simulink model "TermProject_Rectifier"  (R2019a)
settings: Solver=FixedStepDiscrete  StartTime=0.0  StopTime=1  RelTol=1e-3
libraries: powerlib x22, eeGeneralControl x4
settings Model: Creator=ryusl  LastModifiedBy=ryusl

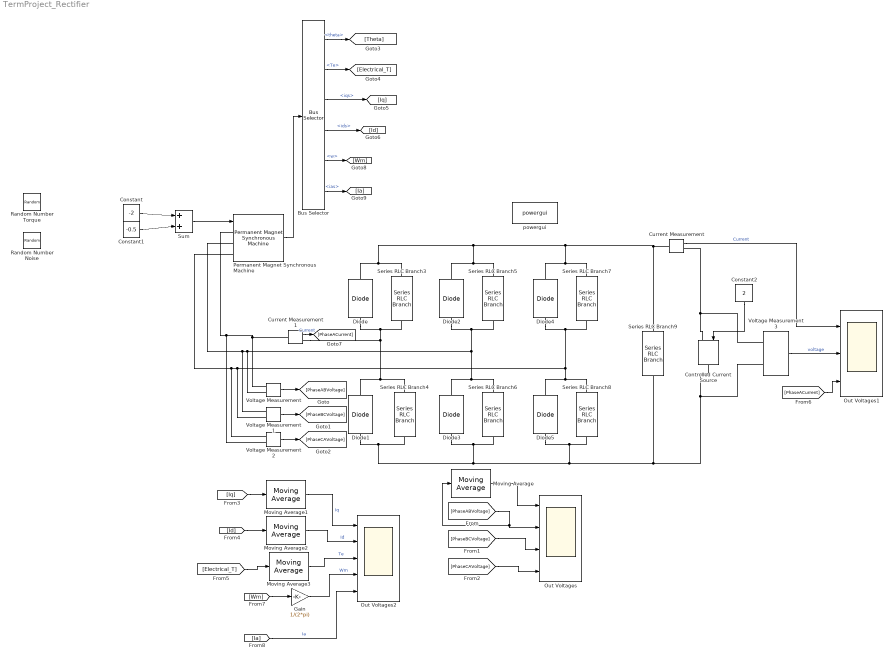
== system TermProject_Rectifier ==
  Bus Selector : BusSelector  OutputSignals=theta,Te,iqs,ids,w,ias
  Constant : Constant  Value=-2
  Constant1 : Constant  Value=-0.5
  Constant2 : Constant  Value=2
  Controlled Current Source : powerlib/Electrical Sources/Controlled Current Source  Initialize=on  Source_Type=AC  Amplitude=0  Phase=0  Frequency=0  Measurements=None
      settings: SourceProductName=Simscape Electrical
  Current Measurement : powerlib/Measurements/Current Measurement  PhasorSimulation=off  OutputType=Complex  PSBequivalent=0
      settings: SourceProductName=Simscape Electrical
  Current Measurement1 : powerlib/Measurements/Current Measurement  PhasorSimulation=off  OutputType=Complex  PSBequivalent=0
      settings: SourceProductName=Simscape Electrical
  Diode{,1..5} (6 alike) : powerlib/Power Electronics/Diode  Ron=0.001  Lon=0  Vf=0  IC=0  UseSnubber=0  Rs=0  Cs=0  Measurements=off
      settings: SourceProductName=Simscape Electrical
  Gain : Gain  Gain=1/(2*pi)
  Moving Average : eeGeneralControl/Moving Average  VariantControl=Variant1  LabelModeActiveChoice=Discrete  f=1000  x0=0  Ts=10e-6
      settings: SourceProductName=Simscape Electrical  SourceProductBaseCode=PS
  Moving Average1 : eeGeneralControl/Moving Average  VariantControl=Variant1  LabelModeActiveChoice=Discrete  f=100  x0=0  Ts=1e-5
      settings: SourceProductName=Simscape Electrical  SourceProductBaseCode=PS
  Moving Average2 : eeGeneralControl/Moving Average  VariantControl=Variant1  LabelModeActiveChoice=Discrete  f=100  x0=0  Ts=1e-5
      settings: SourceProductName=Simscape Electrical  SourceProductBaseCode=PS
  Moving Average3 : eeGeneralControl/Moving Average  VariantControl=Variant1  LabelModeActiveChoice=Discrete  f=100  x0=0  Ts=1e-5
      settings: SourceProductName=Simscape Electrical  SourceProductBaseCode=PS
  Out Voltages : Scope  NumInputPorts=4
  Out Voltages1 : Scope  NumInputPorts=3
  Out Voltages2 : Scope  NumInputPorts=5
  Permanent Magnet Synchronous Machine : powerlib/Machines/Permanent Magnet Synchronous Machine  NbPhases=3  FluxDistribution=Sinusoidal  RotorType=Round  MechanicalLoad=Torque Tm  PresetModel=No  ShowDetailedParameters=on  MeasurementBus=on  Resistance=10.58  Inductance=8.5e-3  dqInductances=[8.5e-3,8.5e-3]  La=16.7e-3  MachineConstant=Voltage Constant (V_peak L-L / krpm)  Flux=0.60646  VoltageCst=110  TorqueCst=0.90969  Flat=120  Mechanical=[0.00027 0.005024 1 0]  PolePairs=4  InitialConditions=[0,0, 0,0]  InitialConditions5ph=[0 0 0 0 0 0]  TsPowergui=0  TsBlock=-1  RefAngle=90 degrees behind phase A axis (modified Park)
  Random Number Noise : RandomNumber  Variance=0.1  SampleTime=1e-3
  Random Number Torque : RandomNumber  Mean=-1.6  Variance=0.05  SampleTime=0.1
  Series RLC Branch{3..8} (6 alike) : powerlib/Elements/Series RLC Branch  LConnTagsString=__new0  RConnTagsString=__new0  BranchType=R  Resistance=1e6  Inductance=1e-3  SetiL0=off  InitialCurrent=0  Capacitance=1e-6  Setx0=off  InitialVoltage=0  Measurements=None
      settings: SourceProductName=Simscape Electrical
  Series RLC Branch9 : powerlib/Elements/Series RLC Branch  LConnTagsString=__new0  RConnTagsString=__new0  BranchType=C  Resistance=1e6  Inductance=1e-3  SetiL0=off  InitialCurrent=0  Capacitance=470e-6  Setx0=off  InitialVoltage=0  Measurements=None
      settings: SourceProductName=Simscape Electrical
  Sum : Sum  Inputs=+|+
  Voltage Measurement{,1..3} (4 alike) : powerlib/Measurements/Voltage Measurement  PhasorSimulation=off  OutputType=Complex  PSBequivalent=0
      settings: SourceProductName=Simscape Electrical
  powergui : powerlib/powergui  Priority=1  SimulationMode=Discrete  SampleTime=1e-6  frequency=60  Iterations=50  frequencyindice=0  Pbase=100e6  ErrMax=1e-4  UnitsV=kV  UnitsW=MW  buscounter=0  FunctionMessages=off  echomessages=off  EnableUseOfTLC=off  CurrentSourceSwitches=off  DisableSnubberDevices=off  DisableRonSwitches=off  DisableVfSwitches=off  DisplayEquations=off  AutomaticDiscreteSolvers=off  SolverType=Tustin/Backward Euler (TBE)  Interpol=off  ExternalGateDelay=off  methode=off  Ts=100  x0status=blocks  SPID=on  SwTol=0  HookPort=off  NonlinearTolerance=0  nMaxIteration=15  ContinueOnMaxIteration=off  RestoreLinks=warning  ResistiveCurrentMeasurement=off  Frange=[0:2:500]  Ylog=off  Xlog=on  ShowGrid=off  save=off  variable=ZData  structure=0  ZoomFFT=off  StartTime=0.0  cycles=1  DisplayStyle=1  fundamental=60  FreqAxis=off  MaxFrequency=1000  frequencyindicesteady=1  RmsSteady=1  display=off
      settings: SourceProductName=Simscape Electrical
  wires:
  Sum/1 -> Permanent Magnet Synchronous Machine/1
  Voltage Measurement/1 -> [PhaseABVoltage]
  Voltage Measurement1/1 -> [PhaseBCVoltage]
  Voltage Measurement2/1 -> [PhaseCAVoltage]
  [PhaseABVoltage] -> Moving Average/1, Out Voltages/2
  [PhaseBCVoltage] -> Out Voltages/3
  [PhaseCAVoltage] -> Out Voltages/4
  Voltage Measurement3/1 -> Out Voltages1/2  "voltage"
  Constant1/1 -> Sum/2
  Constant/1 -> Sum/1
  Moving Average/1 -> Out Voltages/1
  Current Measurement/1 -> Out Voltages1/1  "Current"
  Constant2/1 -> Controlled Current Source/1
  Permanent Magnet Synchronous Machine/1 -> Bus Selector/1
  Bus Selector/1 -> [Theta]  "<theta>"
  Bus Selector/2 -> [Electrical_T]  "<Te>"
  Bus Selector/3 -> [Iq]  "<iqs>"
  Bus Selector/4 -> [Id]  "<ids>"
  [Iq] -> Moving Average1/1
  Moving Average1/1 -> Out Voltages2/1  "Iq"
  [Id] -> Moving Average2/1
  Moving Average2/1 -> Out Voltages2/2  "Id"
  [Electrical_T] -> Moving Average3/1
  Moving Average3/1 -> Out Voltages2/3  "Te"
  Current Measurement1/1 -> [PhaseACurrent]  "Current"
  [PhaseACurrent] -> Out Voltages1/3
  Bus Selector/5 -> [Wm]  "<w>"
  [Wm] -> Gain/1
  Gain/1 -> Out Voltages2/4  "Wm"
  Bus Selector/6 -> [Ia]  "<ias>"
  [Ia] -> Out Voltages2/5  "Ia"
  connections:
  Diode/LConn1 -- Current Measurement1/RConn1 -- Series RLC Branch4/LConn1 -- Diode1/RConn1 -- Series RLC Branch3/RConn1
  Series RLC Branch6/LConn1 -- Permanent Magnet Synchronous Machine/LConn2 -- Voltage Measurement1/LConn1 -- Voltage Measurement/LConn2 -- Diode2/LConn1 -- Series RLC Branch5/RConn1 -- Diode3/RConn1
  Diode/RConn1 -- Series RLC Branch5/LConn1 -- Diode2/RConn1 -- Series RLC Branch9/LConn1 -- Current Measurement/LConn1 -- Series RLC Branch7/LConn1 -- Diode4/RConn1 -- Series RLC Branch3/LConn1
  Diode1/LConn1 -- Series RLC Branch6/RConn1 -- Diode3/LConn1 -- Diode5/LConn1 -- Series RLC Branch8/RConn1 -- Series RLC Branch9/RConn1 -- Controlled Current Source/RConn1 -- Voltage Measurement3/LConn2 -- Series RLC Branch4/RConn1
  Diode5/RConn1 -- Permanent Magnet Synchronous Machine/LConn3 -- Voltage Measurement2/LConn1 -- Voltage Measurement1/LConn2 -- Series RLC Branch7/RConn1 -- Diode4/LConn1 -- Series RLC Branch8/LConn1
  Voltage Measurement3/LConn1 -- Current Measurement/RConn1 -- Controlled Current Source/LConn1
  Permanent Magnet Synchronous Machine/LConn1 -- Voltage Measurement2/LConn2 -- Current Measurement1/LConn1 -- Voltage Measurement/LConn1
